simulink model "gbtspec_mode13"  (Simulink 7.4)
settings: Solver=ode45  StartTime=0.0  StopTime=20000  RelTol=1e-3
libraries: xbsIndex_r4 x265, xps_library x47, dspsigops x16, casper_library_misc x14
(part 1 of 2)
settings Model: Creator=dave  LastModifiedBy=mwagner
settings OptimizationCC: InitFltsAndDblsToZero=on

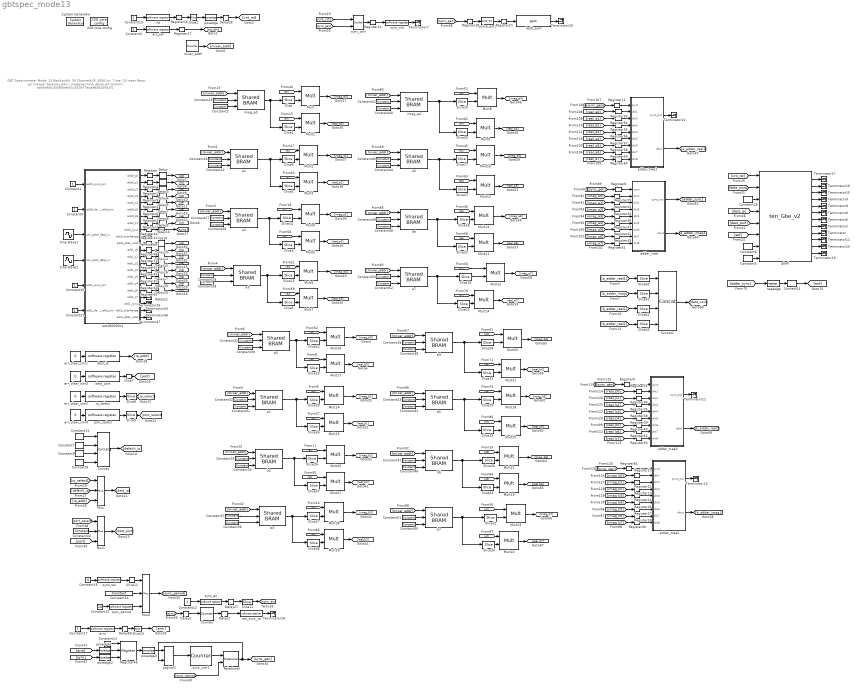
== system gbtspec_mode13 ==
  note: GBT Spectrometer
      | Mode: 13
      | Bandwidth: 30
      | Channels/IF: 4096
      | Int. Time: 10 msec
      | Repo: git://casper.berkeley.edu/~mwagner/mlib_devel.git
      | Commit: ae0be6d1d34f5befa01c913b77ecae840440e2f1
  " System Generator" : xbsIndex_r4/ System Generator  Tag=genX  SystemSampleTime=-1  xilinxfamily=virtex5  part=xc5vsx95t  speed=-1  package=ff1136  synthesis_tool=XST  clock_wrapper=Clock Enables  directory=./gbtspec_mode13/sysgen  testbench=off  simulink_period=1  sysclk_period=6.6667  dcm_input_clock_period=100  incr_netlist=off  trim_vbits=Everywhere in SubSystem  dbl_ovrd=According to Block Masks  core_generation=According to Block Masks  run_coregen=off  deprecated_control=off  eval_field=0  block_type=sysgen
      settings: block_version=10.1.3
  Concat : xbsIndex_r4/Concat  num_inputs=4  dbl_ovrd=off  block_type=concat
  Concat1 : xbsIndex_r4/Concat  num_inputs=4  dbl_ovrd=off  block_type=concat
  Constant{1,4,20..21} (4 alike) : Constant  OutDataType=sfix(16)  OutScaling=2^0  SampleTime=1
  Constant10 : xbsIndex_r4/Constant  arith_type=Unsigned  const=10145  n_bits=32  bin_pt=0  explicit_period=on  period=1  equ=P=C  opselect=C  inp2=PCIN>>17  opr=+  inp1=P  carry=CIN  dbl_ovrd=off  block_type=constant
  Constant11 : xbsIndex_r4/Constant  arith_type=Unsigned  const=10  n_bits=8  bin_pt=0  explicit_period=on  period=1  equ=P=C  opselect=C  inp2=PCIN>>17  opr=+  inp1=P  carry=CIN  dbl_ovrd=off  block_type=constant
  Constant12 : Constant  OutDataType=fixdt(1, 16)  OutScaling=2^0
  Constant13 : xbsIndex_r4/Constant  arith_type=Boolean  const=1  n_bits=16  bin_pt=14  explicit_period=on  period=1  equ=P=C  opselect=C  inp2=PCIN>>17  opr=+  inp1=P  carry=CIN  dbl_ovrd=off  block_type=constant
  Constant14 : xbsIndex_r4/Constant  arith_type=Unsigned  const=100663295  n_bits=32  bin_pt=0  explicit_period=on  period=1  equ=P=C  opselect=C  inp2=PCIN>>17  opr=+  inp1=P  carry=CIN  dbl_ovrd=off  block_type=constant
  Constant15 : Constant  Value=16  OutDataType=sfix(16)  OutScaling=2^0
  Constant16 : Constant  Value=0  OutDataType=sfix(16)  OutScaling=2^0
  Constant17 : Constant  OutDataType=sfix(16)  OutScaling=2^0
  Constant18 : xbsIndex_r4/Constant  arith_type=Boolean  const=1  n_bits=1  bin_pt=0  explicit_period=on  period=1  equ=P=C  opselect=C  inp2=PCIN>>17  opr=+  inp1=P  carry=CIN  dbl_ovrd=off  block_type=constant
  Constant19 : Constant  OutDataType=sfix(16)  OutScaling=2^0
  Constant{2,22,24..53} (32 alike) : xbsIndex_r4/Constant  arith_type=Unsigned  const=0  n_bits=18  bin_pt=0  explicit_period=on  period=1  equ=P=C  opselect=C  inp2=PCIN>>17  opr=+  inp1=P  carry=CIN  dbl_ovrd=off  block_type=constant
  Constant3 : Constant  OutDataType=sfix(16)  OutScaling=2^0
  Constant5 : xbsIndex_r4/Constant  arith_type=Boolean  const=1  n_bits=1  bin_pt=0  explicit_period=on  period=1  equ=P=C  opselect=C  inp2=PCIN>>17  opr=+  inp1=P  carry=CIN  dbl_ovrd=off  block_type=constant
  Constant6 : xbsIndex_r4/Constant  arith_type=Boolean  const=1  n_bits=1  bin_pt=0  explicit_period=on  period=1  equ=P=C  opselect=C  inp2=PCIN>>17  opr=+  inp1=P  carry=CIN  dbl_ovrd=off  block_type=constant
  Constant7 : xbsIndex_r4/Constant  arith_type=Unsigned  const=0  n_bits=8  bin_pt=0  explicit_period=on  period=1  equ=P=C  opselect=C  inp2=PCIN>>17  opr=+  inp1=P  carry=CIN  dbl_ovrd=off  block_type=constant
  Constant8 : xbsIndex_r4/Constant  arith_type=Unsigned  const=0  n_bits=8  bin_pt=0  explicit_period=on  period=1  equ=P=C  opselect=C  inp2=PCIN>>17  opr=+  inp1=P  carry=CIN  dbl_ovrd=off  block_type=constant
  Constant9 : xbsIndex_r4/Constant  arith_type=Unsigned  const=145  n_bits=8  bin_pt=0  explicit_period=on  period=1  equ=P=C  opselect=C  inp2=PCIN>>17  opr=+  inp1=P  carry=CIN  dbl_ovrd=off  block_type=constant
  Convert24 : xbsIndex_r4/Convert  arith_type=Boolean  n_bits=8  bin_pt=6  quantization=Truncate  overflow=Wrap  latency=0  dbl_ovrd=off  pipeline=off  block_type=convert
      settings: xl_area=[0, 0, 0, 0, 0, 0, 0]  block_version=10.1.3
  Counter : xbsIndex_r4/Counter  cnt_type=Free Running  cnt_to=Inf  operation=Up  start_count=0  cnt_by_val=1  arith_type=Unsigned  n_bits=8  bin_pt=0  load_pin=off  rst=off  en=on  explicit_period=on  period=1  dbl_ovrd=off  use_behavioral_HDL=off  implementation=Fabric  block_type=counter
      settings: block_version=11.4
  Delay{,3..5,7..10,13..17,19..21} (16 alike) : xbsIndex_r4/Delay  en=off  latency=3  dbl_ovrd=off  reg_retiming=off  block_type=delay
      settings: block_version=11.4
  Delay1 : xbsIndex_r4/Delay  en=off  latency=8  dbl_ovrd=off  reg_retiming=off  block_type=delay
      settings: block_version=11.4
  Delay2 : xbsIndex_r4/Delay  en=off  latency=8  dbl_ovrd=off  reg_retiming=off  block_type=delay
      settings: block_version=11.4
  Delay26 : xbsIndex_r4/Delay  en=off  latency=8  dbl_ovrd=off  reg_retiming=on  block_type=delay
  Delay27 : xbsIndex_r4/Delay  en=off  latency=8  dbl_ovrd=off  reg_retiming=off  block_type=delay
      settings: block_version=11.4
  Delay60 : xbsIndex_r4/Delay  en=off  latency=2  dbl_ovrd=off  reg_retiming=on  block_type=delay
  Logical1 : xbsIndex_r4/Logical  logical_function=OR  inputs=2  en=off  latency=0  precision=Full  arith_type=Unsigned  n_bits=16  bin_pt=0  align_bp=on  dbl_ovrd=off  block_type=logical
  Mult{,1..31} (32 alike) : xbsIndex_r4/Mult  precision=Full  arith_type="Signed  (2's comp)"  n_bits=16  bin_pt=14  quantization=Truncate  overflow=Wrap  en=off  latency=3  dbl_ovrd=off  use_behavioral_HDL=on  opt=Speed  use_embedded=on  optimum_pipeline=off  pipeline=on  use_rpm=on  placement_style=Triangular  block_type=mult
      settings: block_version=11.4
  Mux : xbsIndex_r4/Mux  inputs=2  en=off  latency=0  precision=Full  arith_type=Unsigned  n_bits=16  bin_pt=14  quantization=Truncate  overflow=Wrap  dbl_ovrd=off  block_type=mux
      settings: block_version=11.4
  Mux1 : xbsIndex_r4/Mux  inputs=2  en=off  latency=0  precision=Full  arith_type=Unsigned  n_bits=16  bin_pt=14  quantization=Truncate  overflow=Wrap  dbl_ovrd=off  block_type=mux
      settings: block_version=11.4
  Mux2 : xbsIndex_r4/Mux  inputs=2  en=off  latency=0  precision=Full  arith_type=Unsigned  n_bits=16  bin_pt=14  quantization=Truncate  overflow=Wrap  dbl_ovrd=off  block_type=mux
      settings: block_version=11.4
  Register{,1..14,16..18,21..24,26..44,46..47,49,51..64} (58 alike) : xbsIndex_r4/Register  init=0  rst=off  en=off  dbl_ovrd=off  block_type=register
      settings: block_version=11.4
  Register45 : xbsIndex_r4/Register  init=0  rst=on  en=on  dbl_ovrd=off  block_type=register
      settings: block_version=11.4
  Relational : xbsIndex_r4/Relational  mode=a>=b  en=off  latency=0  dbl_ovrd=off  block_type=relational
      settings: xl_area=[0, 0, 0, 0, 0, 0, 0]  block_version=9.1.01
  Sine Wave1 : Sin  Amplitude=.9  Bias=0  Frequency=2.*pi/4.  Phase=2*pi*240/200  Samples=10  SampleTime=.0625  Offset=0
  Sine Wave2 : Sin  Amplitude=.9  Bias=0  Frequency=2.*pi/4.  Phase=2*pi*240/200  Samples=10  SampleTime=.0625  Offset=0
  Slice{,6..7,14..19,24,26..31,39..43} (21 alike) : xbsIndex_r4/Slice  nbits=16  boolean_output=off  mode=Lower Bit Location + Width  bit1=0  base1=MSB of Input  bit0=0  base0=LSB of Input  dbl_ovrd=off  block_type=slice
      Slice7 settings: infoedit="Extracts a given range of bits from each input sample and presents it at the output.  The output type is ordinarily unsigned with binary point at zero, but can be Boolean when the slice is one bit wide.<P><P>Hardware notes: In hardware this block costs nothing."  block_version=10.1.3
  Slice{1,3..5,20..23,25,32..38} (16 alike) : xbsIndex_r4/Slice  nbits=16  boolean_output=off  mode=Upper Bit Location + Width  bit1=0  base1=MSB of Input  bit0=0  base0=LSB of Input  dbl_ovrd=off  block_type=slice
  Slice{2,8..13} (7 alike) : xbsIndex_r4/Slice  nbits=1  boolean_output=on  mode=Lower Bit Location + Width  bit1=0  base1=MSB of Input  bit0=0  base0=LSB of Input  dbl_ovrd=off  block_type=slice
      Slice10 settings: infoedit="Extracts a given range of bits from each input sample and presents it at the output.  The output type is ordinarily unsigned with binary point at zero, but can be Boolean when the slice is one bit wide.<P><P>Hardware notes: In hardware this block costs nothing."  block_version=10.1.3
      Slice12 settings: block_version=10.1.3
      Slice13 settings: infoedit="Extracts a given range of bits from each input sample and presents it at the output.  The output type is ordinarily unsigned with binary point at zero, but can be Boolean when the slice is one bit wide.<P><P>Hardware notes: In hardware this block costs nothing."  block_version=10.1.3
      Slice2 settings: block_version=10.1.3
      Slice8 settings: block_version=10.1.3
      Slice9 settings: block_version=10.1.3
  Terminator{,2..3,5..13,15..20,22,26,43,46..47} (23 alike) : Terminator
  XSG core config : xps_library/XSG core config  Tag=xps:xsg  SystemSampleTime=-1  hw_sys=ROACH:sx95t  ibob_linux=off  clk_src=adc0_clk  iBOB_clk_src=adc0_clk  BEE2_ctrl_clk_src=sys_clk  BEE2_usr_clk_src=sys_clk  ROACH_clk_src=adc0_clk  CORR_clk_src=sys_clk  gpio_clk_io_group=iBOB:sma  gpio_clk_bit_index=0  clk_rate=150  sample_period=1  synthesis_tool=XST  mpc_type=powerpc440_ext
  a{1..3,5..7} (6 alike) : xps_library/Shared BRAM  Tag=xps:bram  SystemSampleTime=-1  arith_type="Signed  (2's comp)"  addr_width=11  data_width=32  data_bin_pt=0  init_vals=[1:2^11]  sample_rate=1
  acc_len : xps_library/software register  Tag=xps:sw_reg  SystemSampleTime=-1  io_dir=From Processor  arith_type=Unsigned  bitwidth=32  bin_pt=0  sample_period=1  gw_name=gbtspec_mode13_acc_len_user_data_out
      link override convert: arith_type=Unsigned  n_bits=32  bin_pt=0
      link override r_spec_2048_r102_cnt_rst_user_data_out: arith_type=Unsigned  n_bits=32  bin_pt=0  period=1
      link override r_spec_2048_r102_nosim_cnt_rst_user_data_out: arith_type=Unsigned  n_bits=32  bin_pt=0  period=1
      link override r_spec_2048_r103_cnt_rst_user_data_out: arith_type=Unsigned  n_bits=32  bin_pt=0  period=1
      link override roach_spec_no10gbe_sync_cnt_rst_user_data_out: arith_type=Unsigned  n_bits=32  bin_pt=0  period=1
      link override roach_spec_rst_cnt_user_data_out: arith_type=Unsigned  n_bits=32  bin_pt=0  period=1
      link override roach_spec_rst_sync_cnt_user_data_out: arith_type=Unsigned  n_bits=32  bin_pt=0  period=1
  adc083000x1 : Subsystem  Tag=xps:adc083000x2  AncestorBlock=xps_library/adc083000x2  mask(adc_083000x2){use_adc0=on, use_adc1=on, demux_adc=off, clock_sync=off, verbose=off, using_ctrl=on, adc_clk_rate=600, sample_period=1, bit_width=8}
      mask prompts: use_adc0 "Use ZD0K0?"; use_adc1 "Use ZDOK1?"; demux_adc "Demux ADCs by 2?"; clock_sync "Interleave 2 ADC boards?"; verbose "Verbose Block Creation?"; using_ctrl "Add ports for control registers?"; adc_clk_rate "ADC clock rate (MHz)"; sample_period "Sample Period"; bit_width "Output Bit Width"
      mask help:
      | The ADC block converts analog inputs to digital outputs.
      | Every clock cycle, the inputs are sampled and digitized to
      | 8 bit binary point numbers in the range of [-1, 1).
      |
      | Online block-specific documentation: http://casper.berkeley.edu/wiki/Adc083000
      mask init:
      | adc083000_mask;
      mask Help: eval('xlWeb([getenv(''MLIB_ROOT''), ''\doc\html\sys_adc\sys_adc.html''])')
  adder_tree : Subsystem  AncestorBlock=casper_library_misc/adder_tree  mask(adder_tree){n_inputs=8, latency=1, first_stage_hdl=off, behavioral=on}
      mask prompts: n_inputs "Number of Inputs"; latency "Add Latency"; first_stage_hdl "Use behavioural HDL for first stage of adders"; behavioral "Use behavioral HDL for all adders"
      mask help:
      | Sums all inputs using a tree of adds and delays.
      |
      | Number of inputs: The number of inputs to the block to be summed
      | Add latency: The number of clock cycles to perform one addition (affects timing).
      | Use behavioural HDL for first stage of adders: Causes the first stage of adders to be absorbed into DSP blocks if multipliers precede them (Virtex 5).
      | Use behavioural HDL for all adders: Causes all adders in all stages to be implemented in behavioural HDL (may improve timing).
      mask init:
      | adder_tree_init(gcb, ...
      |     'n_inputs', n_inputs, ...
      |     'latency', latency, ...
      |     'first_stage_hdl', first_stage_hdl, ...
      |     'behavioral', behavioral);
      settings: AttributesFormatString=latency 3
      mask Help: eval('xlWeb(''http://casper.berkeley.edu/wiki/Adder_tree'')')
  adder_tree1 : Subsystem  AncestorBlock=casper_library_misc/adder_tree  mask(adder_tree){n_inputs=8, latency=1, first_stage_hdl=off, behavioral=on}
      mask prompts: n_inputs "Number of Inputs"; latency "Add Latency"; first_stage_hdl "Use behavioural HDL for first stage of adders"; behavioral "Use behavioral HDL for all adders"
      mask help:
      | Sums all inputs using a tree of adds and delays.
      |
      | Number of inputs: The number of inputs to the block to be summed
      | Add latency: The number of clock cycles to perform one addition (affects timing).
      | Use behavioural HDL for first stage of adders: Causes the first stage of adders to be absorbed into DSP blocks if multipliers precede them (Virtex 5).
      | Use behavioural HDL for all adders: Causes all adders in all stages to be implemented in behavioural HDL (may improve timing).
      mask init:
      | adder_tree_init(gcb, ...
      |     'n_inputs', n_inputs, ...
      |     'latency', latency, ...
      |     'first_stage_hdl', first_stage_hdl, ...
      |     'behavioral', behavioral);
      settings: AttributesFormatString=latency 3
      mask Help: eval('xlWeb(''http://casper.berkeley.edu/wiki/Adder_tree'')')
  adder_tree2 : Subsystem  AncestorBlock=casper_library_misc/adder_tree  mask(adder_tree){n_inputs=8, latency=1, first_stage_hdl=off, behavioral=on}
      mask prompts: n_inputs "Number of Inputs"; latency "Add Latency"; first_stage_hdl "Use behavioural HDL for first stage of adders"; behavioral "Use behavioral HDL for all adders"
      mask help:
      | Sums all inputs using a tree of adds and delays.
      |
      | Number of inputs: The number of inputs to the block to be summed
      | Add latency: The number of clock cycles to perform one addition (affects timing).
      | Use behavioural HDL for first stage of adders: Causes the first stage of adders to be absorbed into DSP blocks if multipliers precede them (Virtex 5).
      | Use behavioural HDL for all adders: Causes all adders in all stages to be implemented in behavioural HDL (may improve timing).
      mask init:
      | adder_tree_init(gcb, ...
      |     'n_inputs', n_inputs, ...
      |     'latency', latency, ...
      |     'first_stage_hdl', first_stage_hdl, ...
      |     'behavioral', behavioral);
      settings: AttributesFormatString=latency 3
      mask Help: eval('xlWeb(''http://casper.berkeley.edu/wiki/Adder_tree'')')
  adder_tree3 : Subsystem  AncestorBlock=casper_library_misc/adder_tree  mask(adder_tree){n_inputs=8, latency=1, first_stage_hdl=off, behavioral=on}
      mask prompts: n_inputs "Number of Inputs"; latency "Add Latency"; first_stage_hdl "Use behavioural HDL for first stage of adders"; behavioral "Use behavioral HDL for all adders"
      mask help:
      | Sums all inputs using a tree of adds and delays.
      |
      | Number of inputs: The number of inputs to the block to be summed
      | Add latency: The number of clock cycles to perform one addition (affects timing).
      | Use behavioural HDL for first stage of adders: Causes the first stage of adders to be absorbed into DSP blocks if multipliers precede them (Virtex 5).
      | Use behavioural HDL for all adders: Causes all adders in all stages to be implemented in behavioural HDL (may improve timing).
      mask init:
      | adder_tree_init(gcb, ...
      |     'n_inputs', n_inputs, ...
      |     'latency', latency, ...
      |     'first_stage_hdl', first_stage_hdl, ...
      |     'behavioral', behavioral);
      settings: AttributesFormatString=latency 3
      mask Help: eval('xlWeb(''http://casper.berkeley.edu/wiki/Adder_tree'')')
  arm : xps_library/software register  Tag=xps:sw_reg  SystemSampleTime=-1  io_dir=From Processor  arith_type=Unsigned  bitwidth=32  bin_pt=0  sample_period=1  gw_name=gbtspec_mode13_arm_user_data_out
      link override convert: arith_type=Unsigned  n_bits=32  bin_pt=0
      link override r_spec_2048_r102_cnt_rst_user_data_out: arith_type=Unsigned  n_bits=32  bin_pt=0  period=1
      link override r_spec_2048_r102_nosim_cnt_rst_user_data_out: arith_type=Unsigned  n_bits=32  bin_pt=0  period=1
      link override r_spec_2048_r103_cnt_rst_user_data_out: arith_type=Unsigned  n_bits=32  bin_pt=0  period=1
      link override roach_spec_no10gbe_sync_cnt_rst_user_data_out: arith_type=Unsigned  n_bits=32  bin_pt=0  period=1
      link override roach_spec_rst_cnt_user_data_out: arith_type=Unsigned  n_bits=32  bin_pt=0  period=1
      link override roach_spec_rst_sync_cnt_user_data_out: arith_type=Unsigned  n_bits=32  bin_pt=0  period=1
  b{0..7} (8 alike) : xps_library/Shared BRAM  Tag=xps:bram  SystemSampleTime=-1  arith_type="Signed  (2's comp)"  addr_width=11  data_width=32  data_bin_pt=0  init_vals=[1:2^11]  sample_rate=1
  dest_ip : xps_library/software register  Tag=xps:sw_reg  SystemSampleTime=-1  io_dir=From Processor  arith_type=Unsigned  bitwidth=32  bin_pt=0  sample_period=1  gw_name=gbtspec_mode13_dest_ip_user_data_out
      link override r_10gbe_demo_dest_ip_user_data_out: arith_type=Unsigned  n_bits=32  bin_pt=0  period=1
      link override r_10gbe_test_dest_ip_user_data_out: arith_type=Unsigned  n_bits=32  bin_pt=0  period=1
      link override r_xaui_test_cnt_rst_user_data_out: arith_type=Unsigned  n_bits=32  bin_pt=0  period=1
  dest_port : xps_library/software register  Tag=xps:sw_reg  SystemSampleTime=-1  io_dir=From Processor  arith_type=Unsigned  bitwidth=32  bin_pt=0  sample_period=1  gw_name=gbtspec_mode13_dest_port_user_data_out
      link override r_10gbe_demo_dest_port_user_data_out: arith_type=Unsigned  n_bits=32  bin_pt=0  period=1
      link override r_10gbe_test_dest_port_user_data_out: arith_type=Unsigned  n_bits=32  bin_pt=0  period=1
      link override r_xaui_test_cnt_rst_user_data_out: arith_type=Unsigned  n_bits=32  bin_pt=0  period=1
  err_clear_sim{1..4} (4 alike) : Constant  Value=0  OutDataType=sfix(16)  OutScaling=2^0
  ext_sync_ctr : xps_library/software register  Tag=xps:sw_reg  SystemSampleTime=-1  io_dir=To Processor  arith_type=Unsigned  bitwidth=32  bin_pt=0  sample_period=1  gw_name=gbtspec_mode13_ext_sync_ctr_user_data_in
  gbe0 : xps_library/ten_Gbe_v2  Tag=xps:tengbe_v2  SystemSampleTime=-1  port=0  rx_dist_ram=off  large_frames=off  show_param=off  pre_emph=3  swing=800  fab_en=off  fab_mac=hex2dec('123456780000')  fab_ip=192*(2^24) + 168*(2^16) + 5*(2^8) + 20*(2^0)  fab_udp=10000  fab_gate=1  cpu_rx_en=on  cpu_tx_en=on
  imag_a0 : xps_library/Shared BRAM  Tag=xps:bram  SystemSampleTime=-1  arith_type="Signed  (2's comp)"  addr_width=11  data_width=32  data_bin_pt=0  init_vals=[1:2^11]  sample_rate=1
  imag_a4 : xps_library/Shared BRAM  Tag=xps:bram  SystemSampleTime=-1  arith_type="Signed  (2's comp)"  addr_width=11  data_width=32  data_bin_pt=0  init_vals=[1:2^11]  sample_rate=1
  ip_select : xps_library/software register  Tag=xps:sw_reg  SystemSampleTime=-1  io_dir=From Processor  arith_type=Unsigned  bitwidth=32  bin_pt=0  sample_period=1  gw_name=gbtspec_mode13_ip_select_user_data_out
      link override r_10gbe_demo_gbe_core_rst_user_data_out: arith_type=Unsigned  n_bits=32  bin_pt=0  period=1
      link override r_10gbe_test_cnt_rst_user_data_out: arith_type=Unsigned  n_bits=32  bin_pt=0  period=1
      link override r_10gbe_test_gbe_core_rst_user_data_out: arith_type=Unsigned  n_bits=32  bin_pt=0  period=1
      link override r_xaui_test_cnt_rst_user_data_out: arith_type=Unsigned  n_bits=32  bin_pt=0  period=1
  led0_sync : xps_library/gpio  Tag=xps:gpio  SystemSampleTime=-1  io_group=ROACH:led  io_dir=out  arith_type=Boolean  bitwidth=1  bin_pt=0  bit_index=0  sample_period=1  use_single_ended=off  use_ddr=off  reg_iob=on  reg_clk_phase=0  termination=None
      link override convert: arith_type=Boolean  n_bits=1  bin_pt=0
  mixer_addr : xbsIndex_r4/Counter  cnt_type=Free Running  cnt_to=Inf  operation=Up  start_count=0  cnt_by_val=1  arith_type=Unsigned  n_bits=8  bin_pt=0  load_pin=off  rst=off  en=off  explicit_period=on  period=1  dbl_ovrd=off  use_behavioral_HDL=off  implementation=Fabric  block_type=counter
      settings: block_version=11.4
  negedge : casper_library_misc/negedge  Tag=Rising Edge Detector  SystemSampleTime=-1
  port_select : xps_library/software register  Tag=xps:sw_reg  SystemSampleTime=-1  io_dir=From Processor  arith_type=Unsigned  bitwidth=32  bin_pt=0  sample_period=1  gw_name=gbtspec_mode13_port_select_user_data_out
      link override r_10gbe_demo_gbe_core_rst_user_data_out: arith_type=Unsigned  n_bits=32  bin_pt=0  period=1
      link override r_10gbe_test_cnt_rst_user_data_out: arith_type=Unsigned  n_bits=32  bin_pt=0  period=1
      link override r_10gbe_test_gbe_core_rst_user_data_out: arith_type=Unsigned  n_bits=32  bin_pt=0  period=1
      link override r_xaui_test_cnt_rst_user_data_out: arith_type=Unsigned  n_bits=32  bin_pt=0  period=1
  posedge{,1..3} (4 alike) : casper_library_misc/posedge  Tag=Rising Edge Detector  SystemSampleTime=-1
  pulse_ext1 : casper_library_misc/pulse_ext  SystemSampleTime=-1  pulse_len=2^24
  rst : xps_library/software register  Tag=xps:sw_reg  SystemSampleTime=-1  io_dir=From Processor  arith_type=Unsigned  bitwidth=32  bin_pt=0  sample_period=1  gw_name=gbtspec_mode13_rst_user_data_out
      link override convert: arith_type=Unsigned  n_bits=32  bin_pt=0
      link override r_spec_2048_r102_cnt_rst_user_data_out: arith_type=Unsigned  n_bits=32  bin_pt=0  period=1
      link override r_spec_2048_r102_nosim_cnt_rst_user_data_out: arith_type=Unsigned  n_bits=32  bin_pt=0  period=1
      link override r_spec_2048_r103_cnt_rst_user_data_out: arith_type=Unsigned  n_bits=32  bin_pt=0  period=1
      link override roach_spec_no10gbe_sync_cnt_rst_user_data_out: arith_type=Unsigned  n_bits=32  bin_pt=0  period=1
      link override roach_spec_rst_cnt_user_data_out: arith_type=Unsigned  n_bits=32  bin_pt=0  period=1
      link override roach_spec_rst_sync_cnt_user_data_out: arith_type=Unsigned  n_bits=32  bin_pt=0  period=1
  sync_cnt : xps_library/software register  Tag=xps:sw_reg  SystemSampleTime=-1  io_dir=To Processor  arith_type=Unsigned  bitwidth=32  bin_pt=0  sample_period=1  gw_name=gbtspec_mode13_sync_cnt_user_data_in
      link override convert: arith_type=Unsigned  n_bits=32  bin_pt=0
      link override r_spec_2048_r102_cnt_rst_user_data_out: arith_type=Unsigned  n_bits=32  bin_pt=0  period=1
      link override r_spec_2048_r102_nosim_cnt_rst_user_data_out: arith_type=Unsigned  n_bits=32  bin_pt=0  period=1
      link override r_spec_2048_r103_cnt_rst_user_data_out: arith_type=Unsigned  n_bits=32  bin_pt=0  period=1
      link override roach_spec_no10gbe_sync_cnt_rst_user_data_out: arith_type=Unsigned  n_bits=32  bin_pt=0  period=1
      link override roach_spec_rst_cnt_user_data_out: arith_type=Unsigned  n_bits=32  bin_pt=0  period=1
      link override roach_spec_rst_sync_cnt_user_data_out: arith_type=Unsigned  n_bits=32  bin_pt=0  period=1
  sync_cntr : xbsIndex_r4/Counter  cnt_type=Free Running  cnt_to=Inf  operation=Up  start_count=0  cnt_by_val=1  arith_type=Unsigned  n_bits=32  bin_pt=0  load_pin=off  rst=on  en=on  explicit_period=on  period=1  dbl_ovrd=off  use_behavioral_HDL=off  implementation=Fabric  use_rpm=off  block_type=counter
  sync_cntr1 : xbsIndex_r4/Counter  cnt_type=Free Running  cnt_to=1023  operation=Up  start_count=0  cnt_by_val=1  arith_type=Unsigned  n_bits=10  bin_pt=0  load_pin=off  rst=on  en=off  explicit_period=on  period=1  dbl_ovrd=off  use_behavioral_HDL=off  implementation=Fabric  use_rpm=on  block_type=counter
      settings: xl_area=[0, 0, 0, 0, 0, 0, 0]  block_version=9.1.01
  sync_en : xps_library/software register  Tag=xps:sw_reg  SystemSampleTime=-1  io_dir=From Processor  arith_type=Unsigned  bitwidth=32  bin_pt=0  sample_period=1  gw_name=gbtspec_mode13_sync_en_user_data_out
  sync_period : xps_library/software register  Tag=xps:sw_reg  SystemSampleTime=-1  io_dir=From Processor  arith_type=Unsigned  bitwidth=32  bin_pt=0  sample_period=1  gw_name=gbtspec_mode13_sync_period_user_data_out
      link override convert: arith_type=Unsigned  n_bits=32  bin_pt=0
      link override r_spec_2048_r102_cnt_rst_user_data_out: arith_type=Unsigned  n_bits=32  bin_pt=0  period=1
      link override r_spec_2048_r102_nosim_cnt_rst_user_data_out: arith_type=Unsigned  n_bits=32  bin_pt=0  period=1
      link override r_spec_2048_r103_cnt_rst_user_data_out: arith_type=Unsigned  n_bits=32  bin_pt=0  period=1
      link override roach_spec_no10gbe_sync_cnt_rst_user_data_out: arith_type=Unsigned  n_bits=32  bin_pt=0  period=1
      link override roach_spec_rst_cnt_user_data_out: arith_type=Unsigned  n_bits=32  bin_pt=0  period=1
      link override roach_spec_rst_sync_cnt_user_data_out: arith_type=Unsigned  n_bits=32  bin_pt=0  period=1
  sync_sel : xps_library/software register  Tag=xps:sw_reg  SystemSampleTime=-1  io_dir=From Processor  arith_type=Unsigned  bitwidth=32  bin_pt=0  sample_period=1  gw_name=gbtspec_mode13_sync_sel_user_data_out
      link override convert: arith_type=Unsigned  n_bits=32  bin_pt=0
      link override r_spec_2048_r102_cnt_rst_user_data_out: arith_type=Unsigned  n_bits=32  bin_pt=0  period=1
      link override r_spec_2048_r102_nosim_cnt_rst_user_data_out: arith_type=Unsigned  n_bits=32  bin_pt=0  period=1
      link override r_spec_2048_r103_cnt_rst_user_data_out: arith_type=Unsigned  n_bits=32  bin_pt=0  period=1
      link override roach_spec_no10gbe_sync_cnt_rst_user_data_out: arith_type=Unsigned  n_bits=32  bin_pt=0  period=1
      link override roach_spec_rst_cnt_user_data_out: arith_type=Unsigned  n_bits=32  bin_pt=0  period=1
      link override roach_spec_rst_sync_cnt_user_data_out: arith_type=Unsigned  n_bits=32  bin_pt=0  period=1
  wires:
  led0_sync/1 -> Terminator20/1
  pulse_ext1/1 -> Register21/1
  sync_cntr/1 -> Register14/1
  rst/1 -> Register16/1
  Constant19/1 -> rst/1
  sync_cnt/1 -> Terminator7/1
  Constant3/1 -> acc_len/1
  acc_len/1 -> Register17/1
  Register16/1 -> Slice2/1
  Register14/1 -> sync_cnt/1
  [cnt_rst] -> sync_cntr/1
  Slice2/1 -> posedge/1
  [sync_gen] -> Register18/1
  [sync_gen] -> sync_cntr/2
  Register17/1 -> [acc_len]
  Register21/1 -> led0_sync/1
  Register18/1 -> pulse_ext1/1
  Register/1 -> Delay/1
  Constant4/1 -> adc083000x1/2(adc0_data_valid_sim)
  Sine Wave1/1 -> adc083000x1/3(sim_adc0_data_in)
  Constant1/1 -> adc083000x1/1(adc0_sync_sim)
  Constant6/1 -> gbe0/7
  [dest_port] -> gbe0/5
  [cnt_rst] -> gbe0/1
  gbe0/9 -> Terminator/1
  gbe0/1 -> Terminator17/1
  gbe0/2 -> Terminator16/1
  gbe0/3 -> Terminator15/1
  gbe0/4 -> Terminator9/1
  gbe0/5 -> Terminator8/1
  gbe0/6 -> Terminator6/1
  gbe0/7 -> Terminator5/1
  gbe0/8 -> Terminator2/1
  gbe0/10 -> Terminator11/1
  gbe0/11 -> Terminator10/1
  gbe0/12 -> Terminator19/1
  err_clear_sim1/1 -> dest_ip/1
  dest_ip/1 -> [ip_addr]
  dest_port/1 -> Slice7/1
  [dest_ip] -> gbe0/4
  err_clear_sim3/1 -> dest_port/1
  Slice7/1 -> [port]
  Constant5/1 -> gbe0/8
  Constant11/1 -> Concat/1
  Constant7/1 -> Concat/2
  Constant8/1 -> Concat/3
  Constant9/1 -> Concat/4
  Concat/1 -> [default_ip]
  [default_ip] -> Mux/2
  Mux/1 -> [dest_ip]
  [ip_addr] -> Mux/3
  err_clear_sim2/1 -> ip_select/1
  ip_select/1 -> Slice8/1
  Slice8/1 -> [ip_select]
  [ip_select] -> Mux/1
  Constant10/1 -> Mux1/2
  Mux1/1 -> [dest_port]
  [port] -> Mux1/3
  [port_select] -> Mux1/1
  err_clear_sim4/1 -> port_select/1
  port_select/1 -> Slice9/1
  Slice9/1 -> [port_select]
  [eof] -> gbe0/6
  [data_sout] -> gbe0/2
  Slice10/1 -> [sync]
  Register44/1 -> Slice10/1
  Constant12/1 -> sync_en/1
  sync_en/1 -> Delay27/1
  Slice11/1 -> [sync_en]
  Delay27/1 -> Slice11/1
  Counter/1 -> Delay2/1
  [sync] -> Delay1/1
  ext_sync_ctr/1 -> Terminator18/1
  Delay1/1 -> Counter/1
  Delay2/1 -> ext_sync_ctr/1
  Mux2/1 -> [sync_period]
  Constant15/1 -> sync_period/1
  sync_period/1 -> Mux2/3
  Constant14/1 -> Mux2/2
  sync_sel/1 -> Slice12/1
  Constant16/1 -> sync_sel/1
  Slice12/1 -> Mux2/1
  Constant13/1 -> Register45/1
  posedge1/1 -> Register45/2
  Register45/1 -> posedge3/1
  posedge3/1 -> Logical1/1
  Logical1/1 -> sync_cntr1/1
  sync_cntr1/1 -> Relational/1
  Relational/1 -> [sync_gen], Logical1/2
  [arm] -> posedge1/1
  Constant17/1 -> arm/1
  Delay60/1 -> Slice13/1
  arm/1 -> Delay60/1
  Slice13/1 -> [arm]
  [sync] -> posedge2/1
  posedge2/1 -> Register45/3
  [sync_period] -> Relational/2
  adc083000x1/9(adc0_sync) -> Register44/1
  adc083000x1/20(adc1_sync) -> Terminator43/1
  adc083000x1/21(adc1_outofrange) -> Terminator46/1
  adc083000x1/22(adc1_data_valid) -> Terminator47/1
  negedge/1 -> Convert24/1
  Convert24/1 -> [eof]
  [adder_sync] -> negedge/1
  posedge/1 -> Delay26/1
  Sine Wave2/1 -> adc083000x1/4(sim_adc1_data_in)
  Constant20/1 -> adc083000x1/5(adc1_sync_sim)
  Constant21/1 -> adc083000x1/6(adc1_data_valid_sim)
  Delay26/1 -> [cnt_rst]
  adc083000x1/1(adc0_s0) -> Register/1
  adc083000x1/3(adc0_s2) -> Register1/1
  adc083000x1/5(adc0_s4) -> Register2/1
  adc083000x1/7(adc0_s6) -> Register3/1
  adc083000x1/12(adc1_s0) -> Register46/1
  adc083000x1/14(adc1_s2) -> Register47/1
  adc083000x1/16(adc1_s5) -> Register52/1
  adc083000x1/17(adc1_s4) -> Register43/1
  adc083000x1/18(adc1_s6) -> Register61/1
  adc083000x1/19(adc1_s7) -> Terminator26/1
  adc083000x1/8(adc0_s7) -> Register7/1
  Register7/1 -> Delay10/1
  Register3/1 -> Delay9/1
  Register6/1 -> Delay8/1
  adc083000x1/6(adc0_s5) -> Register6/1
  Register2/1 -> Delay7/1
  Register5/1 -> Delay5/1
  Register1/1 -> Delay4/1
  Register4/1 -> Delay3/1
  adc083000x1/2(adc0_s1) -> Register4/1
  adc083000x1/4(adc0_s3) -> Register5/1
  adc083000x1/10(adc0_outofrange) -> Terminator3/1
  adc083000x1/13(adc1_s1) -> Register13/1
  adc083000x1/11(adc0_data_valid) -> Register12/1
  adc083000x1/15(adc1_s3) -> Register42/1
  Register12/1 -> Delay13/1
  Register46/1 -> Delay14/1
  Register13/1 -> Delay15/1
  Register47/1 -> Delay16/1
  Register42/1 -> Delay17/1
  Register52/1 -> Delay19/1
  Register43/1 -> Delay20/1
  Register61/1 -> Delay21/1
  mixer_addr/1 -> [mixer_addr]
  [mixer_addr] -> imag_a0/1
  Constant2/1 -> imag_a0/3
  Constant25/1 -> imag_a0/2
  [a0] -> Mult/1
  imag_a0/1 -> Slice/1, Slice1/1
  [a0] -> Mult1/1
  Mult/1 -> [imag_a0]
  Mult1/1 -> [real_a0]
  [a1] -> Mult2/1
  a1/1 -> Slice6/1, Slice3/1
  [a1] -> Mult3/1
  Mult2/1 -> [imag_a1]
  Mult3/1 -> [real_a1]
  [a2] -> Mult4/1
  [a2] -> Mult5/1
  Mult4/1 -> [imag_a2]
  Mult5/1 -> [real_a2]
  [a3] -> Mult6/1
  [a3] -> Mult7/1
  Mult6/1 -> [imag_a3]
  Mult7/1 -> [real_a3]
  a2/1 -> Slice14/1, Slice4/1
  a3/1 -> Slice15/1, Slice5/1
  [mixer_addr] -> imag_a4/1
  Constant40/1 -> imag_a4/3
  Constant41/1 -> imag_a4/2
  [a4] -> Mult8/1
  imag_a4/1 -> Slice16/1, Slice20/1
  [a4] -> Mult9/1
  Mult8/1 -> [imag_a4]
  Mult9/1 -> [real_a4]
  [mixer_addr] -> a5/1
  Constant44/1 -> a5/3
  Constant45/1 -> a5/2
  [a5] -> Mult10/1
  a5/1 -> Slice17/1, Slice21/1
  [a5] -> Mult12/1
  Mult10/1 -> [imag_a5]
  Mult12/1 -> [real_a5]
  [mixer_addr] -> a6/1
  Constant48/1 -> a6/3
  Constant49/1 -> a6/2
  [a6] -> Mult13/1
  [a6] -> Mult11/1
  Mult13/1 -> [imag_a6]
  Mult11/1 -> [real_a6]
  [mixer_addr] -> a7/1
  Constant52/1 -> a7/3
  Constant53/1 -> a7/2
  [a7] -> Mult15/1
  [a7] -> Mult14/1
  Mult15/1 -> [imag_a7]
  Mult14/1 -> [real_a7]
  a6/1 -> Slice18/1, Slice22/1
  a7/1 -> Slice19/1, Slice23/1
  [sync_gen] -> Register8/1
  Register8/1 -> adder_tree/1(sync)
  [imag_a1] -> Register32/1
  [imag_a0] -> Register29/1
  [imag_a2] -> Register33/1
  [imag_a3] -> Register36/1
  [imag_a4] -> Register37/1
  [imag_a5] -> Register41/1
  [imag_a6] -> Register49/1
  [imag_a7] -> Register51/1
  [sync_gen] -> Register11/1
  Register11/1 -> adder_tree1/1(sync)
  [real_a1] -> Register54/1
  [real_a0] -> Register53/1
  [real_a2] -> Register55/1
  [real_a4] -> Register56/1
  [real_a4] -> Register57/1
  [real_a5] -> Register58/1
  [real_a6] -> Register59/1
  [real_a7] -> Register60/1
  adder_tree1/2(dout) -> [a_adder_real1]
  adder_tree/2(dout) -> [a_adder_imag1]
  adder_tree/1(sync_out) -> [adder_sync]
  adder_tree1/1(sync_out) -> Terminator22/1
  Delay/1 -> [a0]
  Delay3/1 -> [a1]
  Delay4/1 -> [a2]
  Delay5/1 -> [a3]
  Delay7/1 -> [a4]
  Delay8/1 -> [a5]
  Delay9/1 -> [a6]
  Delay10/1 -> [a7]
  Delay13/1 -> [b0]
  Delay14/1 -> [b1]
  Delay15/1 -> [b2]
  Delay16/1 -> [b3]
  Delay17/1 -> [b4]
  Delay19/1 -> [b5]
  Delay20/1 -> [b6]
  Delay21/1 -> [b7]
  Register29/1 -> adder_tree/2(din1)
  Register32/1 -> adder_tree/3(din2)
  Register33/1 -> adder_tree/4(din3)
  Register36/1 -> adder_tree/5(din4)
  Register37/1 -> adder_tree/6(din5)
  Register41/1 -> adder_tree/7(din6)
  Register49/1 -> adder_tree/8(din7)
  Register51/1 -> adder_tree/9(din8)
  Register53/1 -> adder_tree1/2(din1)
  Register54/1 -> adder_tree1/3(din2)
  Register55/1 -> adder_tree1/4(din3)
  Register56/1 -> adder_tree1/5(din4)
  Register57/1 -> adder_tree1/6(din5)
  Register58/1 -> adder_tree1/7(din6)
  Register59/1 -> adder_tree1/8(din7)
  Register60/1 -> adder_tree1/9(din8)
  Slice/1 -> Mult/2
  Slice1/1 -> Mult1/2
  Slice6/1 -> Mult2/2
  Slice3/1 -> Mult3/2
  Slice14/1 -> Mult4/2
  Slice4/1 -> Mult5/2
  Slice15/1 -> Mult6/2
  Slice5/1 -> Mult7/2
  Slice16/1 -> Mult8/2
  Slice20/1 -> Mult9/2
  Slice17/1 -> Mult10/2
  Slice21/1 -> Mult12/2
  Slice18/1 -> Mult13/2
  Slice22/1 -> Mult11/2
  Slice23/1 -> Mult14/2
  Constant24/1 -> a1/2
  Constant22/1 -> a1/3
  Constant27/1 -> a2/2
  Constant26/1 -> a2/3
  Constant29/1 -> a3/2
  Constant28/1 -> a3/3
  [mixer_addr] -> a1/1
  [mixer_addr] -> a2/1
  [mixer_addr] -> a3/1
  [mixer_addr] -> b0/1
  Constant30/1 -> b0/3
  Constant33/1 -> b0/2
  [a0] -> Mult16/1
  b0/1 -> Slice25/1, Slice24/1
  [a0] -> Mult17/1
  Mult16/1 -> [imag_b0]
  Mult17/1 -> [real_b0]
  [a1] -> Mult24/1
  b1/1 -> Slice36/1, Slice39/1
  [a1] -> Mult25/1
  Mult24/1 -> [imag_b1]
  Mult25/1 -> [real_b1]
  [a2] -> Mult26/1
  [a2] -> Mult27/1
  Mult26/1 -> [imag_b2]
  Mult27/1 -> [real_b2]
  [a3] -> Mult28/1
  [a3] -> Mult29/1
  Mult28/1 -> [imag_b3]
  Mult29/1 -> [real_b3]
  b2/1 -> Slice37/1, Slice26/1
  b3/1 -> Slice38/1, Slice27/1
  [mixer_addr] -> b4/1
  Constant38/1 -> b4/3
  Constant39/1 -> b4/2
  [a4] -> Mult30/1
  b4/1 -> Slice32/1, Slice28/1
  [a4] -> Mult31/1
  Mult30/1 -> [imag_b4]
  Mult31/1 -> [real_b4]
  [mixer_addr] -> b5/1
  Constant42/1 -> b5/3
  Constant43/1 -> b5/2
  [a5] -> Mult18/1
  b5/1 -> Slice33/1, Slice29/1
  [a5] -> Mult20/1
  Mult18/1 -> [imag_b5]
  Mult20/1 -> [real_b5]
  [mixer_addr] -> b6/1
  Constant46/1 -> b6/3
  Constant47/1 -> b6/2
  [a6] -> Mult21/1
  [a6] -> Mult19/1
  Mult21/1 -> [imag_b6]
  Mult19/1 -> [real_b6]
  [mixer_addr] -> b7/1
  Constant50/1 -> b7/3
  Constant51/1 -> b7/2
  [a7] -> Mult23/1
  [a7] -> Mult22/1
  Mult23/1 -> [imag_b7]
  Mult22/1 -> [real_b7]
  b6/1 -> Slice34/1, Slice30/1
  b7/1 -> Slice35/1, Slice31/1
  Slice24/1 -> Mult16/2
  Slice25/1 -> Mult17/2
  Slice39/1 -> Mult24/2
  Slice36/1 -> Mult25/2
  Slice26/1 -> Mult26/2
  Slice37/1 -> Mult27/2
  Slice27/1 -> Mult28/2
  Slice38/1 -> Mult29/2
  Slice28/1 -> Mult30/2
  Slice32/1 -> Mult31/2
  Slice29/1 -> Mult18/2
  Slice33/1 -> Mult20/2
  Slice30/1 -> Mult21/2
  Slice34/1 -> Mult19/2
  Slice35/1 -> Mult22/2
  Constant32/1 -> b1/2
  Constant31/1 -> b1/3
  Constant35/1 -> b2/2
  Constant34/1 -> b2/3
  Constant37/1 -> b3/2
  Constant36/1 -> b3/3
  [mixer_addr] -> b1/1
  [mixer_addr] -> b2/1
  [mixer_addr] -> b3/1
  [sync_gen] -> Register64/1
  Register64/1 -> adder_tree2/1(sync)
  [imag_b1] -> Register22/1
  [imag_b0] -> Register10/1
  [imag_b2] -> Register23/1
  [imag_b3] -> Register24/1
  [imag_b4] -> Register26/1
  [imag_b5] -> Register27/1
  [imag_b6] -> Register28/1
  [imag_b7] -> Register30/1
  [sync_gen] -> Register9/1
  Register9/1 -> adder_tree3/1(sync)
  [real_b1] -> Register34/1
  [real_b0] -> Register31/1
  [real_b2] -> Register35/1
  [real_b3] -> Register38/1
  [real_b4] -> Register39/1
  [real_b5] -> Register40/1
  [real_b6] -> Register62/1
  [real_b7] -> Register63/1
  adder_tree3/2(dout) -> [b_adder_real1]
  adder_tree2/2(dout) -> [b_adder_imag1]
  adder_tree2/1(sync_out) -> Terminator13/1
  adder_tree3/1(sync_out) -> Terminator12/1
  Register10/1 -> adder_tree2/2(din1)
  Register22/1 -> adder_tree2/3(din2)
  Register23/1 -> adder_tree2/4(din3)
  Register24/1 -> adder_tree2/5(din4)
  Register26/1 -> adder_tree2/6(din5)
  Register27/1 -> adder_tree2/7(din6)
  Register28/1 -> adder_tree2/8(din7)
  Register30/1 -> adder_tree2/9(din8)
  Register31/1 -> adder_tree3/2(din1)
  Register34/1 -> adder_tree3/3(din2)
  Register35/1 -> adder_tree3/4(din3)
  Register38/1 -> adder_tree3/5(din4)
  Register39/1 -> adder_tree3/6(din5)
  Register40/1 -> adder_tree3/7(din6)
  Register62/1 -> adder_tree3/8(din7)
  Register63/1 -> adder_tree3/9(din8)
  [a_adder_real1] -> Slice40/1
  Slice40/1 -> Concat1/1
  Slice41/1 -> Concat1/2
  Slice42/1 -> Concat1/3
  Slice43/1 -> Concat1/4
  [a_adder_imag1] -> Slice41/1
  [b_adder_real1] -> Slice42/1
  [b_adder_real1] -> Slice43/1
  Concat1/1 -> [data_sout]
  Slice19/1 -> Mult15/2
  Slice31/1 -> Mult23/2
  Constant18/1 -> gbe0/3
